simulink model "Motormodell"  (R2021a)
settings: Solver=VariableStepAuto  StartTime=0.0  StopTime=10.0  RelTol=1e-3
undefined symbols (not defined in the file or in its folder): J, k3, k4, ks, L, R, Ua
settings Model: Creator=johannes  LastModifiedBy=johannes

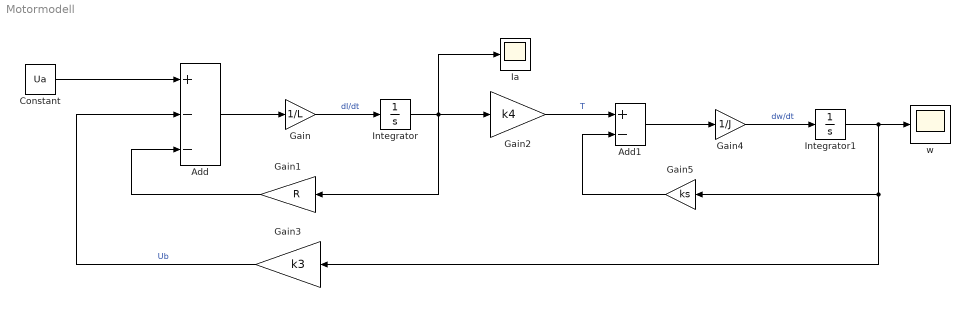
== system Motormodell ==
  Add : Sum  Inputs=+--
  Add1 : Sum  Inputs=+-
  Constant : Constant  Value=Ua
  Gain : Gain  Gain=1/L
  Gain1 : Gain  Gain=R
  Gain2 : Gain  Gain=k4
  Gain3 : Gain  Gain=k3
  Gain4 : Gain  Gain=1/J
  Gain5 : Gain  Gain=ks
  Ia : Scope
  Integrator : Integrator
  Integrator1 : Integrator
  w : Scope
  wires:
  Constant/1 -> Add/1
  Integrator/1 -> Ia/1, Gain2/1, Gain1/1
  Gain/1 -> Integrator/1  "dI/dt"
  Add/1 -> Gain/1
  Gain3/1 -> Add/2  "Ub"
  Gain1/1 -> Add/3
  Integrator1/1 -> w/1, Gain5/1, Gain3/1
  Gain4/1 -> Integrator1/1  "dw/dt"
  Gain2/1 -> Add1/1  "T"
  Add1/1 -> Gain4/1
  Gain5/1 -> Add1/2
